simulink model "SpeedgoatCANOpen2Buses100us"  (R2018b)
settings: Solver=FixedStepDiscrete  StartTime=0.0  StopTime=inf  FixedStep=0.0001  RelTol=1e-3  EnableMultiTasking=on
libraries: slrtlib x6, speedgoatlib_IO691 x5, simulink x3, dspstat3 x2, cstblocks x1
(part 2 of 2)

== system SpeedgoatCANOpen2Buses100us/Speedgoat_TPDOs/CAN Bus Communication/CANOpen Slave Protocol Stack - CAN Bus #2 (B) ==
  C Caller : CCaller  FunctionName=CANOpenSlave_ProcessStack_APT  PortSpecificationStruct="%)30     .    ( D   8    (     @         %    \"     8    !     0         %  0 \"0    $    V    07)G3F%M90  4&]R=$YA;64 4V-O<&4     26YD97@     5'EP90      4VEZ90         .    ,     8    (    !          %    \"     $    $     0         0  0 <GA)1 X    P    !@    @    $          4    (     0    0    !         !  ! !R>$E$#@   #@    &    \"     0         !0    @    !    !0    $         $     4   !);G ...(+2763 chars)"
  CAN RX Wrapper : Subsystem
  CAN TX Wrapper : Subsystem
  wires:
  CAN RX Wrapper/3(DATA) -> C Caller/3
  C Caller/3 -> CAN TX Wrapper/3(DATA)
  CAN RX Wrapper/2(DLC) -> C Caller/2
  C Caller/1 -> CAN TX Wrapper/1(ID)
  CAN RX Wrapper/1(ID) -> C Caller/1
  C Caller/2 -> CAN TX Wrapper/2(DLC), CAN TX Wrapper/Enable

== system SpeedgoatCANOpen2Buses100us/Trike Application Layer/System_Control/BrakeControl ==
  Brake control [%] : Inport
  Amp2mAmp : Gain  Gain=1000
  Data Type Conversion : DataTypeConversion  OutDataTypeStr=uint16
  Gain1 : Gain  Gain=12.7
  Gain2 : Gain  Gain=-1
  Gain3 : Gain  Gain=0.00015625
  Saturation : Saturate  UpperLimit=0  LowerLimit=-1
  Saturation1 : Saturate  UpperLimit=10000  LowerLimit=3600
  Sum : Sum  Inputs=|+-
  offset : Constant  Value=3600
  Br CurrentRef [mA] : Outport
  wires:
  Saturation/1 -> Gain1/1
  Gain1/1 -> Amp2mAmp/1
  Brake control [%]/1 -> Data Type Conversion/1
  Gain2/1 -> Saturation/1
  Amp2mAmp/1 -> Br CurrentRef [mA]/1  "Br CurrentRef"
  Sum/1 -> Gain3/1
  offset/1 -> Sum/2
  Gain3/1 -> Gain2/1  "br_percent"
  Data Type Conversion/1 -> Saturation1/1
  Saturation1/1 -> Sum/1

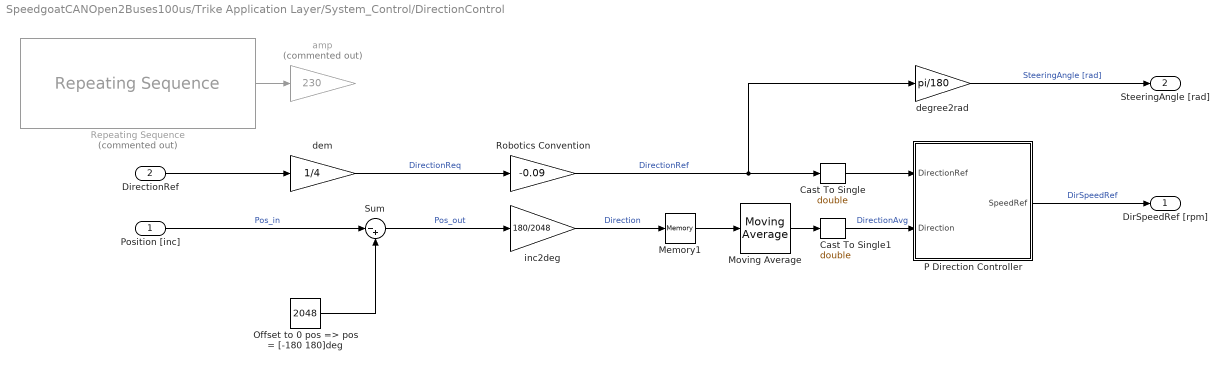
== system SpeedgoatCANOpen2Buses100us/Trike Application Layer/System_Control/DirectionControl ==
  Position [inc] : Inport
  DirectionRef : Inport  Port=2
  Cast To Single : DataTypeConversion  OutDataTypeStr=double
  Cast To Single1 : DataTypeConversion  OutDataTypeStr=double
  Memory1 : Memory  InheritSampleTime=on
  Moving Average : dspstat3/Moving Average  Method=Sliding window  ForgettingFactorPort=off  SpecifyWindowLength=on  WindowLength=1  ForgettingFactor=0.9  SimulateUsing=Code generation
  Offset to 0 pos => pos = [-180 180]deg : Constant  Value=2048
  P Direction Controller : MATLAB Function  TreatAsAtomicUnit=on  SystemSampleTime=5e-3
  Repeating Sequence : simulink/Sources/Repeating Sequence  Commented=on  rep_seq_t=[0 3 3.01 6 6.01 9 9.01 12]*5  rep_seq_y=[1 1 0 0 -1 -1 0 0]
  Robotics Convention : Gain  Gain=-0.09
  Sum : Sum  Inputs=|-+
  amp : Gain  Commented=on  Gain=230
  degree2rad : Gain  Gain=pi/180
  dem : Gain  Gain=1/4
  inc2deg : Gain  Gain=180/2048
  DirSpeedRef [rpm] : Outport
  SteeringAngle [rad] : Outport  Port=2
  wires:
  Memory1/1 -> Moving Average/1
  degree2rad/1 -> SteeringAngle [rad]/1  "SteeringAngle [rad]"
  inc2deg/1 -> Memory1/1  "Direction"
  DirectionRef/1 -> dem/1
  P Direction Controller/1(SpeedRef) -> DirSpeedRef [rpm]/1  "DirSpeedRef"
  Robotics Convention/1 -> Cast To Single/1, degree2rad/1  "DirectionRef"
  Cast To Single/1 -> P Direction Controller/1(DirectionRef)
  Cast To Single1/1 -> P Direction Controller/2(Direction)  "DirectionAvg"
  Position [inc]/1 -> Sum/1  "Pos_in"
  Sum/1 -> inc2deg/1  "Pos_out"
  Offset to 0 pos => pos = [-180 180]deg/1 -> Sum/2
  Moving Average/1 -> Cast To Single1/1
  Repeating Sequence/1 -> amp/1
  dem/1 -> Robotics Convention/1  "DirectionReq"

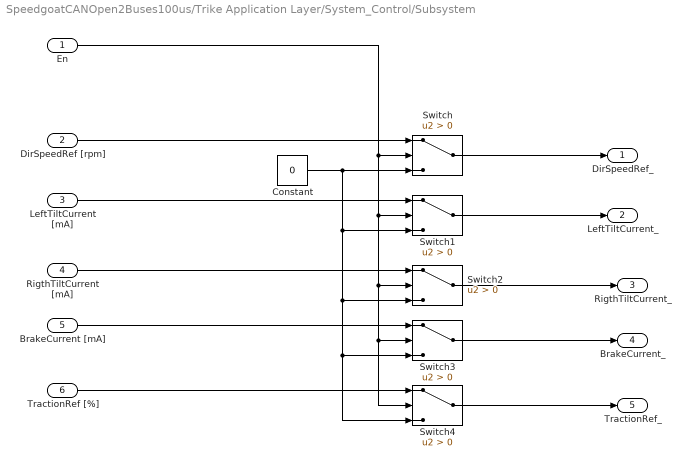
== system SpeedgoatCANOpen2Buses100us/Trike Application Layer/System_Control/Subsystem ==
  En : Inport
  DirSpeedRef [rpm] : Inport  Port=2
  LeftTiltCurrent [mA] : Inport  Port=3
  RigthTiltCurrent [mA] : Inport  Port=4
  BrakeCurrent [mA] : Inport  Port=5
  TractionRef [%] : Inport  Port=6
  Constant : Constant  Value=0
  Switch{,1..4} (5 alike) : Switch  Criteria=u2 > Threshold
  DirSpeedRef_ : Outport
  LeftTiltCurrent_ : Outport  Port=2
  RigthTiltCurrent_ : Outport  Port=3
  BrakeCurrent_ : Outport  Port=4
  TractionRef_ : Outport  Port=5
  wires:
  TractionRef [%]/1 -> Switch4/1
  Switch1/1 -> LeftTiltCurrent_/1
  Switch2/1 -> RigthTiltCurrent_/1
  En/1 -> Switch1/2, Switch2/2, Switch3/2, Switch4/2, Switch/2
  DirSpeedRef [rpm]/1 -> Switch/1
  LeftTiltCurrent [mA]/1 -> Switch1/1
  Constant/1 -> Switch3/3, Switch4/3, Switch2/3, Switch1/3, Switch/3
  Switch/1 -> DirSpeedRef_/1
  BrakeCurrent [mA]/1 -> Switch3/1
  Switch3/1 -> BrakeCurrent_/1
  Switch4/1 -> TractionRef_/1
  RigthTiltCurrent [mA]/1 -> Switch2/1

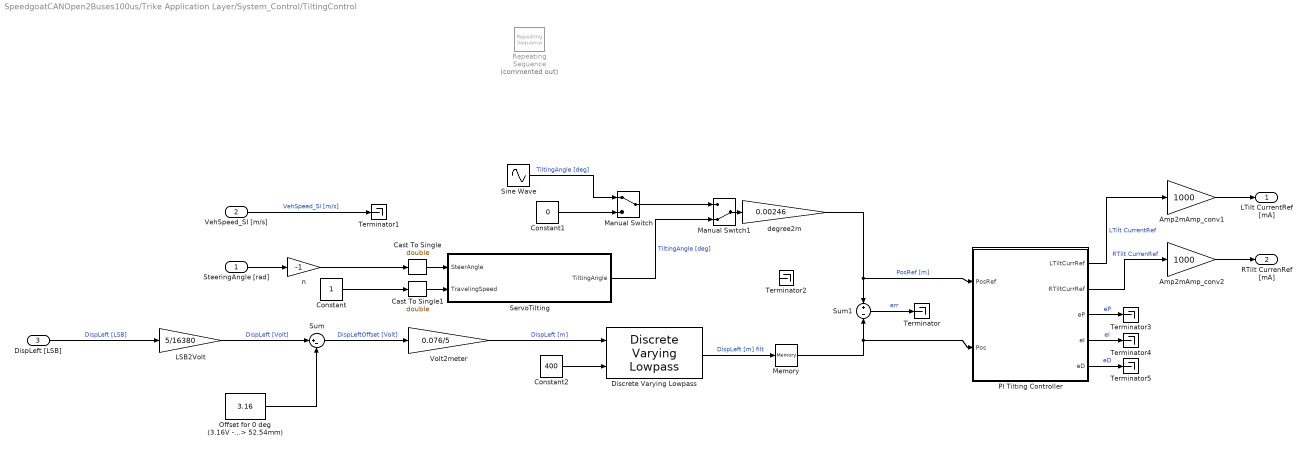
== system SpeedgoatCANOpen2Buses100us/Trike Application Layer/System_Control/TiltingControl ==
  SteeringAngle [rad] : Inport
  VehSpeed_SI [m/s] : Inport  Port=2
  DispLeft [LSB] : Inport  Port=3
  Amp2mAmp_conv1 : Gain  Gain=1000
  Amp2mAmp_conv2 : Gain  Gain=1000
  Cast To Single : DataTypeConversion  OutDataTypeStr=double
  Cast To Single1 : DataTypeConversion  OutDataTypeStr=double
  Constant : Constant
  Constant1 : Constant  Value=0
  Constant2 : Constant  Value=400
  Discrete Varying Lowpass : cstblocks/Linear Parameter Varying/Discrete Varying Lowpass  N=1  w0=0.5  Ts=0.0001
      settings: SourceProductName=Control System Toolbox  SourceProductBaseCode=CT
  LSB2Volt : Gain  Gain=5/16380
  Manual Switch : ManualSwitch
  Manual Switch1 : ManualSwitch  CurrentSetting=0
  Memory : Memory  InheritSampleTime=on
  "Offset for 0 deg (3.16V -> 52.54mm)" : Constant  Value=3.16
  PI Tilting Controller : MATLAB Function  TreatAsAtomicUnit=on  SystemSampleTime=5e-3
  Repeating Sequence : simulink/Sources/Repeating Sequence  Commented=on  rep_seq_t=[0 10 10.01 20 20.01 30 30.01 40] * 0.004  rep_seq_y=[1 1 -1 -1 1 1 -1 -1]
  ServoTilting : MATLAB Function  TreatAsAtomicUnit=on
      settings: MinAlgLoopOccurrences=on
  Sine Wave : Sin  Amplitude=2  Frequency=0.5  SampleTime=0
  Sum : Sum  Inputs=|+-
  Sum1 : Sum  Inputs=+-
  Terminator{,1..5} (6 alike) : Terminator
  Volt2meter : Gain  Gain=0.076/5
  degree2m : Gain  Gain=0.00246
  n : Gain  Gain=-1
  LTilt CurrentRef [mA] : Outport
  RTilt CurrenRef [mA] : Outport  Port=2
  wires:
  degree2m/1 -> Sum1/1, PI Tilting Controller/1(PosRef)  "PosRef [m]"
  Memory/1 -> PI Tilting Controller/2(Pos), Sum1/2
  Sine Wave/1 -> Manual Switch/1  "TiltingAngle [deg]"
  SteeringAngle [rad]/1 -> n/1
  Volt2meter/1 -> Discrete Varying Lowpass/1  "DispLeft [m]"
  PI Tilting Controller/2(RTiltCurrRef) -> Amp2mAmp_conv2/1  "RTilt CurrenRef"
  "Offset for 0 deg (3.16V -> 52.54mm)"/1 -> Sum/2
  PI Tilting Controller/1(LTiltCurrRef) -> Amp2mAmp_conv1/1  "LTilt CurrentRef"
  Constant/1 -> Cast To Single1/1
  Cast To Single/1 -> ServoTilting/1(SteerAngle)
  Cast To Single1/1 -> ServoTilting/2(TravelingSpeed)
  DispLeft [LSB]/1 -> LSB2Volt/1  "DispLeft [LSB]"
  Amp2mAmp_conv1/1 -> LTilt CurrentRef [mA]/1
  Amp2mAmp_conv2/1 -> RTilt CurrenRef [mA]/1
  Sum/1 -> Volt2meter/1  "DispLeftOffset [Volt]"
  Sum1/1 -> Terminator/1  "err"
  VehSpeed_SI [m/s]/1 -> Terminator1/1  "VehSpeed_SI [m/s]"
  Constant1/1 -> Manual Switch/2
  ServoTilting/1(TiltingAngle) -> Manual Switch1/2  "TiltingAngle [deg]"
  LSB2Volt/1 -> Sum/1  "DispLeft [Volt]"
  Discrete Varying Lowpass/1 -> Memory/1  "DispLeft [m] filt"
  Constant2/1 -> Discrete Varying Lowpass/2
  Manual Switch/1 -> Manual Switch1/1
  PI Tilting Controller/3(eP) -> Terminator3/1  "eP"
  PI Tilting Controller/4(eI) -> Terminator4/1  "eI"
  PI Tilting Controller/5(eD) -> Terminator5/1  "eD"
  Manual Switch1/1 -> degree2m/1
  n/1 -> Cast To Single/1

== system SpeedgoatCANOpen2Buses100us/Trike Application Layer/System_Control/TractionControl ==
  Traction Torque [%] : Inport
  SpeedRear_Fb : Inport  Port=2
  Abs : Abs
  Gain1 : Gain  Gain=1/10
  Gain2 : Gain  Gain=pi/30
  Terminator1 : Terminator
  WheelRadius : Gain  Gain=0.25
  m/s2Km/h : Gain  Gain=3.6
  VehSpeed_SI [m/s] : Outport
  TractionRef [%] : Outport  Port=2
  wires:
  Traction Torque [%]/1 -> Gain1/1
  Abs/1 -> TractionRef [%]/1  "TractionRef"
  WheelRadius/1 -> m/s2Km/h/1, VehSpeed_SI [m/s]/1  "VehSpeed_SI"
  SpeedRear_Fb/1 -> Gain2/1
  Gain2/1 -> WheelRadius/1  "SpeedRear_SI"
  m/s2Km/h/1 -> Terminator1/1  "VehSpeed_Km/h"
  Gain1/1 -> Abs/1

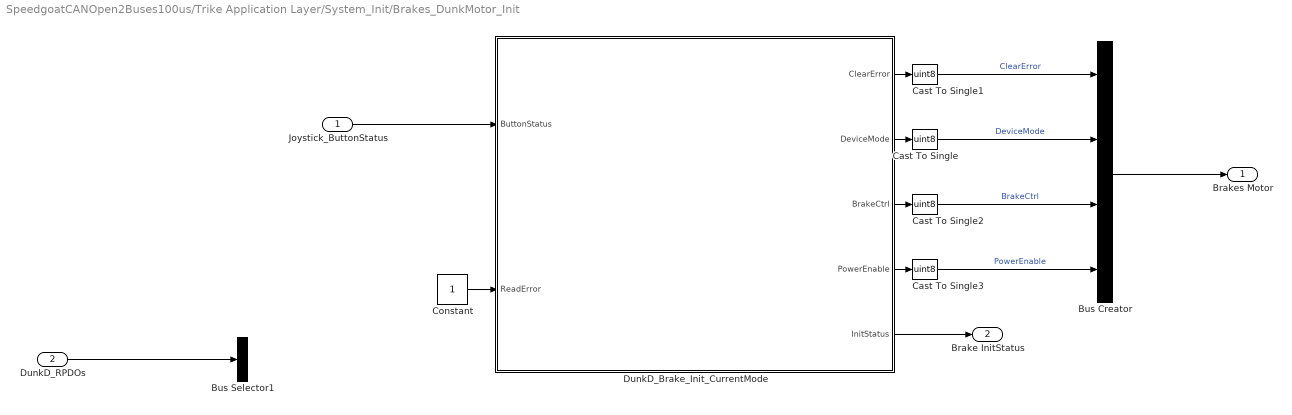
== system SpeedgoatCANOpen2Buses100us/Trike Application Layer/System_Init/Brakes_DunkMotor_Init ==
  Joystick_ButtonStatus : Inport
  DunkD_RPDOs : Inport  Port=2  OutDataTypeStr=Bus: Dunk_RPDOs
  Bus Creator : BusCreator  Inputs=4  OutDataTypeStr=Bus: Dunk_Init_TPDOs
  Bus Selector1 : BusSelector  OutputSignals=DunkD_ActualVelocity
  Cast To Single{,1..3} (4 alike) : DataTypeConversion  OutDataTypeStr=uint8
  Constant : Constant  OutDataTypeStr=single
  DunkD_Brake_Init_CurrentMode : Stateflow chart  TreatAsAtomicUnit=on
  Brakes Motor : Outport  OutDataTypeStr=Bus: Dunk_Init_TPDOs
  Brake InitStatus : Outport  Port=2
  wires:
  DunkD_RPDOs/1 -> Bus Selector1/1
  Bus Creator/1 -> Brakes Motor/1
  Cast To Single1/1 -> Bus Creator/1  "ClearError"
  Cast To Single/1 -> Bus Creator/2  "DeviceMode"
  Cast To Single2/1 -> Bus Creator/3  "BrakeCtrl"
  Cast To Single3/1 -> Bus Creator/4  "PowerEnable"
  DunkD_Brake_Init_CurrentMode/5(InitStatus) -> Brake InitStatus/1
  DunkD_Brake_Init_CurrentMode/1(ClearError) -> Cast To Single1/1
  Joystick_ButtonStatus/1 -> DunkD_Brake_Init_CurrentMode/1(ButtonStatus)
  DunkD_Brake_Init_CurrentMode/2(DeviceMode) -> Cast To Single/1
  DunkD_Brake_Init_CurrentMode/3(BrakeCtrl) -> Cast To Single2/1
  DunkD_Brake_Init_CurrentMode/4(PowerEnable) -> Cast To Single3/1
  Constant/1 -> DunkD_Brake_Init_CurrentMode/2(ReadError)

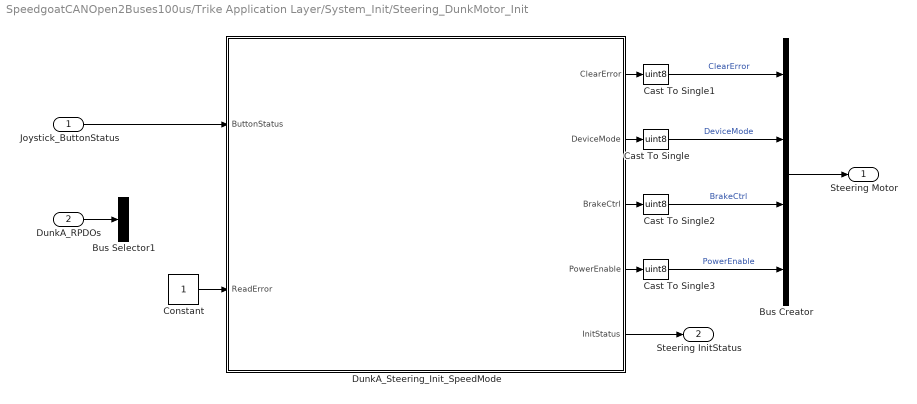
== system SpeedgoatCANOpen2Buses100us/Trike Application Layer/System_Init/Steering_DunkMotor_Init ==
  Joystick_ButtonStatus : Inport
  DunkA_RPDOs : Inport  Port=2  OutDataTypeStr=Bus: Dunk_RPDOs
  Bus Creator : BusCreator  Inputs=4  OutDataTypeStr=Bus: Dunk_Init_TPDOs
  Bus Selector1 : BusSelector  OutputSignals=DunkA_ActualVelocity
  Cast To Single{,1..3} (4 alike) : DataTypeConversion  OutDataTypeStr=uint8
  Constant : Constant  OutDataTypeStr=single
  DunkA_Steering_Init_SpeedMode : Stateflow chart  TreatAsAtomicUnit=on
  Steering Motor : Outport  OutDataTypeStr=Bus: Dunk_Init_TPDOs
  Steering InitStatus : Outport  Port=2
  wires:
  Bus Creator/1 -> Steering Motor/1
  DunkA_RPDOs/1 -> Bus Selector1/1
  DunkA_Steering_Init_SpeedMode/1(ClearError) -> Cast To Single1/1
  DunkA_Steering_Init_SpeedMode/2(DeviceMode) -> Cast To Single/1
  DunkA_Steering_Init_SpeedMode/3(BrakeCtrl) -> Cast To Single2/1
  DunkA_Steering_Init_SpeedMode/4(PowerEnable) -> Cast To Single3/1
  Joystick_ButtonStatus/1 -> DunkA_Steering_Init_SpeedMode/1(ButtonStatus)
  Constant/1 -> DunkA_Steering_Init_SpeedMode/2(ReadError)
  Cast To Single1/1 -> Bus Creator/1  "ClearError"
  Cast To Single/1 -> Bus Creator/2  "DeviceMode"
  Cast To Single2/1 -> Bus Creator/3  "BrakeCtrl"
  Cast To Single3/1 -> Bus Creator/4  "PowerEnable"
  DunkA_Steering_Init_SpeedMode/5(InitStatus) -> Steering InitStatus/1

== system SpeedgoatCANOpen2Buses100us/Trike Application Layer/System_Init/Subsystem ==
  Steering InitStatus : Inport
  TiltLeft InitStatus : Inport  Port=2
  TiltRight InitStatus : Inport  Port=3
  Brake InitStatus : Inport  Port=4
  MiniMaster_Enable : Inport  Port=5
  Compare To Constant : simulink/Logic and Bit Operations/Compare To Constant  relop===  const=5  OutDataTypeStr=boolean
  Sum : Sum  Inputs=+++++
  EnableControl : Outport
  wires:
  Sum/1 -> Compare To Constant/1
  Brake InitStatus/1 -> Sum/4  "Brake_InitStatus"
  Steering InitStatus/1 -> Sum/1  "Steering_InitStatus"
  TiltRight InitStatus/1 -> Sum/3  "TiltRight_InitStatus"
  TiltLeft InitStatus/1 -> Sum/2  "TiltLeft_InitStatus"
  MiniMaster_Enable/1 -> Sum/5  "MiniMaster_Enable"
  Compare To Constant/1 -> EnableControl/1  "EnableControl"

== system SpeedgoatCANOpen2Buses100us/Trike Application Layer/System_Init/TiltingLeft_DunkMotor_Init ==
  Joystick_ButtonStatus : Inport
  DunkB_RPDOs : Inport  Port=2  OutDataTypeStr=Bus: Dunk_RPDOs
  Bus Creator : BusCreator  Inputs=4  OutDataTypeStr=Bus: Dunk_Init_TPDOs
  Bus Selector1 : BusSelector  OutputSignals=DunkB_ActualVelocity
  Cast To Single{,1..3} (4 alike) : DataTypeConversion  OutDataTypeStr=uint8
  Constant : Constant  OutDataTypeStr=single
  DunkB_TiltLeft_Init_CurrentMode : Stateflow chart  TreatAsAtomicUnit=on
  TiltLeft Motor : Outport  OutDataTypeStr=Bus: Dunk_Init_TPDOs
  TiltLeft InitStatus : Outport  Port=2
  wires:
  DunkB_RPDOs/1 -> Bus Selector1/1
  Bus Creator/1 -> TiltLeft Motor/1
  DunkB_TiltLeft_Init_CurrentMode/5(InitStatus) -> TiltLeft InitStatus/1
  Cast To Single/1 -> Bus Creator/2  "DeviceMode"
  Constant/1 -> DunkB_TiltLeft_Init_CurrentMode/2(ReadError)
  Cast To Single2/1 -> Bus Creator/3  "BrakeCtrl"
  DunkB_TiltLeft_Init_CurrentMode/4(PowerEnable) -> Cast To Single3/1
  DunkB_TiltLeft_Init_CurrentMode/3(BrakeCtrl) -> Cast To Single2/1
  Cast To Single3/1 -> Bus Creator/4  "PowerEnable"
  DunkB_TiltLeft_Init_CurrentMode/2(DeviceMode) -> Cast To Single/1
  Cast To Single1/1 -> Bus Creator/1  "ClearError"
  DunkB_TiltLeft_Init_CurrentMode/1(ClearError) -> Cast To Single1/1
  Joystick_ButtonStatus/1 -> DunkB_TiltLeft_Init_CurrentMode/1(ButtonStatus)

== system SpeedgoatCANOpen2Buses100us/Trike Application Layer/System_Init/TiltingRight_DunkMotor_Init ==
  Joystick_ButtonStatus : Inport
  DunkC_RPDOs : Inport  Port=2  OutDataTypeStr=Bus: Dunk_RPDOs
  Bus Creator : BusCreator  Inputs=4  OutDataTypeStr=Bus: Dunk_Init_TPDOs
  Bus Selector1 : BusSelector  OutputSignals=DunkC_ActualVelocity
  Cast To Single{,1..3} (4 alike) : DataTypeConversion  OutDataTypeStr=uint8
  Constant : Constant  OutDataTypeStr=single
  DunkC_TiltRight_Init_CurrentMode : Stateflow chart  TreatAsAtomicUnit=on
  TiltRight Motor : Outport  OutDataTypeStr=Bus: Dunk_Init_TPDOs
  TiltRight InitStatus : Outport  Port=2
  wires:
  Bus Creator/1 -> TiltRight Motor/1
  DunkC_RPDOs/1 -> Bus Selector1/1
  Cast To Single1/1 -> Bus Creator/1  "ClearError"
  Cast To Single/1 -> Bus Creator/2  "DeviceMode"
  Cast To Single2/1 -> Bus Creator/3  "BrakeCtrl"
  Cast To Single3/1 -> Bus Creator/4  "PowerEnable"
  DunkC_TiltRight_Init_CurrentMode/5(InitStatus) -> TiltRight InitStatus/1
  DunkC_TiltRight_Init_CurrentMode/1(ClearError) -> Cast To Single1/1
  Joystick_ButtonStatus/1 -> DunkC_TiltRight_Init_CurrentMode/1(ButtonStatus)
  DunkC_TiltRight_Init_CurrentMode/2(DeviceMode) -> Cast To Single/1
  DunkC_TiltRight_Init_CurrentMode/3(BrakeCtrl) -> Cast To Single2/1
  DunkC_TiltRight_Init_CurrentMode/4(PowerEnable) -> Cast To Single3/1
  Constant/1 -> DunkC_TiltRight_Init_CurrentMode/2(ReadError)

== system SpeedgoatCANOpen2Buses100us/Speedgoat_TPDOs/CAN Bus Communication/CANOpen Slave Protocol Stack - CAN Bus #1 (A)/CAN RX Wrapper ==
  CAN Read : speedgoatlib_IO691/CAN Read  id=1  ts=Ts  channel=1  messageType=RAW  canType=CAN (HS)  initValues=[691 1 0.0001 0 2 1]
      settings: SourceProductName=Simulink Real-Time: Speedgoat Library
  Constant : Constant  Commented=on  Value=0  OutDataTypeStr=Inherit: Inherit via back propagation
  Switch : Switch  Criteria=u2 > Threshold
  Terminator : Terminator
  Terminator1 : Terminator
  ID : Outport
  DLC : Outport  Port=2
  DATA : Outport  Port=3
  wires:
  CAN Read/4 -> Switch/3
  CAN Read/5 -> Terminator1/1
  Switch/1 -> DLC/1
  CAN Read/2 -> ID/1
  CAN Read/3 -> Switch/2
  CAN Read/6 -> DATA/1
  Constant/1 -> Switch/1
  CAN Read/1 -> Terminator/1

== system SpeedgoatCANOpen2Buses100us/Speedgoat_TPDOs/CAN Bus Communication/CANOpen Slave Protocol Stack - CAN Bus #1 (A)/CAN TX Wrapper ==
  ID : Inport
  DLC : Inport  Port=2
  DATA : Inport  Port=3
  Enable : EnablePort
  CAN Write : speedgoatlib_IO691/CAN Write  id=1  ts=Ts  channel=1  messageType=RAW  enableStatusPort=off  canType=CAN (HS)  initValues=[691 1 0.0001 0 2 1 0]
      settings: SourceProductName=Simulink Real-Time: Speedgoat Library
  Constant : Constant  Value=0  OutDataTypeStr=Inherit: Inherit via back propagation
  wires:
  ID/1 -> CAN Write/1
  DATA/1 -> CAN Write/4
  DLC/1 -> CAN Write/3
  Constant/1 -> CAN Write/2

== system SpeedgoatCANOpen2Buses100us/Speedgoat_TPDOs/CAN Bus Communication/CANOpen Slave Protocol Stack - CAN Bus #2 (B)/CAN RX Wrapper ==
  CAN Read : speedgoatlib_IO691/CAN Read  id=1  ts=Ts  channel=2  messageType=RAW  canType=CAN (HS)  initValues=[691 1 0.0001 1 2 1]
      settings: SourceProductName=Simulink Real-Time: Speedgoat Library
  Constant : Constant  Commented=on  Value=0  OutDataTypeStr=Inherit: Inherit via back propagation
  Switch : Switch  Criteria=u2 > Threshold
  Terminator : Terminator
  Terminator1 : Terminator
  ID : Outport
  DLC : Outport  Port=2
  DATA : Outport  Port=3
  wires:
  CAN Read/1 -> Terminator/1
  Constant/1 -> Switch/1
  CAN Read/6 -> DATA/1
  CAN Read/3 -> Switch/2
  CAN Read/2 -> ID/1
  Switch/1 -> DLC/1
  CAN Read/5 -> Terminator1/1
  CAN Read/4 -> Switch/3

== system SpeedgoatCANOpen2Buses100us/Speedgoat_TPDOs/CAN Bus Communication/CANOpen Slave Protocol Stack - CAN Bus #2 (B)/CAN TX Wrapper ==
  ID : Inport
  DLC : Inport  Port=2
  DATA : Inport  Port=3
  Enable : EnablePort
  CAN Write : speedgoatlib_IO691/CAN Write  id=1  ts=Ts  channel=2  messageType=RAW  enableStatusPort=off  canType=CAN (HS)  initValues=[691 1 0.0001 1 2 1 0]
      settings: SourceProductName=Simulink Real-Time: Speedgoat Library
  Constant : Constant  Value=0  OutDataTypeStr=Inherit: Inherit via back propagation
  wires:
  Constant/1 -> CAN Write/2
  DLC/1 -> CAN Write/3
  DATA/1 -> CAN Write/4
  ID/1 -> CAN Write/1

== stateflow chart SpeedgoatCANOpen2Buses100us/Trike Application Layer/System_Init/TiltingLeft_DunkMotor_Init/DunkB_TiltLeft_Init_CurrentMode ==
  state Init
    entry:
    ClearError       = 0;
    DeviceMode   = 0;
    BrakeCtrl        = 0;
    PowerEnable = 0;
    aux                 = 0;
    InitStatus        = 0;
  state Clear_Error
    du:
    ClearError = 1;
    aux=aux+1;
    InitStatus = 0;
  state Wait
    en:
    BrakeCtrl = 2;
    aux = 0;
    InitStatus = 0;
  state SetCurrentMode
    du:
    DeviceMode  = 2;
    PowerEnable = 1;
    InitStatus       = 1;
  (default) -> Init
  Init -> Clear_Error : [ButtonStatus == 1 || ReadError ~= 1]
  Wait -> Init [order 3] : [ReadError ~= 1]
  SetCurrentMode -> Init : [ReadError ~= 1]
  Clear_Error -> Wait : [aux>2000]
  Wait -> Wait [order 1] : [ButtonStatus==0 && ReadError == 1]
  Wait -> SetCurrentMode [order 2] : [ButtonStatus==2 && ReadError == 1]
  data: ButtonStatus input single; ClearError output single; DeviceMode output single; BrakeCtrl output single; ReadError input single; aux2 local single; aux local single; PowerEnable output single; InitStatus output single

== stateflow chart SpeedgoatCANOpen2Buses100us/Trike Application Layer/System_Init/TiltingRight_DunkMotor_Init/DunkC_TiltRight_Init_CurrentMode ==
  state Init
    entry:
    ClearError       = 0;
    DeviceMode   = 0;
    BrakeCtrl        = 0;
    PowerEnable = 0;
    aux                 = 0;
    InitStatus        = 0;
  state Clear_Error
    du:
    ClearError = 1;
    aux=aux+1;
    InitStatus = 0;
  state Wait
    en:
    BrakeCtrl = 2;
    aux = 0;
    InitStatus = 0;
  state SetCurrentMode
    du:
    DeviceMode  = 2;
    PowerEnable = 1;
    InitStatus       = 1;
  (default) -> Init
  Init -> Clear_Error : [ButtonStatus == 1 || ReadError ~= 1]
  Wait -> Init [order 3] : [ReadError ~= 1]
  SetCurrentMode -> Init : [ReadError ~= 1]
  Clear_Error -> Wait : [aux>2000]
  Wait -> Wait [order 1] : [ButtonStatus==0 && ReadError == 1]
  Wait -> SetCurrentMode [order 2] : [ButtonStatus==2 && ReadError == 1]
  data: ButtonStatus input single; ClearError output single; DeviceMode output single; BrakeCtrl output single; ReadError input single; aux2 local single; aux local single; PowerEnable output single; InitStatus output single

== stateflow chart SpeedgoatCANOpen2Buses100us/Trike Application Layer/System_Init/Brakes_DunkMotor_Init/DunkD_Brake_Init_CurrentMode ==
  state Init
    entry:
    ClearError       = 0;
    DeviceMode   = 0;
    BrakeCtrl        = 0;
    PowerEnable = 0;
    aux                 = 0;
    InitStatus        = 0;
  state Clear_Error
    du:
    ClearError = 1;
    aux=aux+1;
    InitStatus = 0;
  state Wait
    en:
    BrakeCtrl = 2;
    aux = 0;
    InitStatus = 0;
  state SetCurrentMode
    du:
    DeviceMode  = 2;
    PowerEnable = 1;
    InitStatus       = 1;
  (default) -> Init
  Init -> Clear_Error : [ButtonStatus == 1 || ReadError ~= 1]
  Wait -> Init [order 3] : [ReadError ~= 1]
  SetCurrentMode -> Init : [ReadError ~= 1]
  Clear_Error -> Wait : [aux>2000]
  Wait -> Wait [order 1] : [ButtonStatus==0 && ReadError == 1]
  Wait -> SetCurrentMode [order 2] : [ButtonStatus==2 && ReadError == 1]
  data: ButtonStatus input single; ClearError output single; DeviceMode output single; BrakeCtrl output single; ReadError input single; aux2 local single; aux local single; PowerEnable output single; InitStatus output single

== stateflow chart SpeedgoatCANOpen2Buses100us/Trike Application Layer/System_Init/EnableCtrl ==
  state Init
    du:
    Enable    =  0;
  state Enable_Control
    du:
    Enable    =  1;
  (default) -> Init
  Init -> Enable_Control : [ButtonStatus == 6 ]
  Enable_Control -> Init : [ButtonStatus == 7 ]
  data: ButtonStatus input single; Enable output single

== matlab function SpeedgoatCANOpen2Buses100us/Trike Application Layer/System_Control/DirectionControl/P Direction Controller ==
  data: DirectionRef input; SpeedRef output; Direction input
function SpeedRef  = fcn(DirectionRef,Direction)


if (DirectionRef>90)
    DirectionRef=90;
end
if (DirectionRef<-90)
    DirectionRef=-90;
end
err = DirectionRef - Direction;

Kp = 70;

SpeedRef = Kp * err;  


end

== matlab function SpeedgoatCANOpen2Buses100us/Trike Application Layer/System_Control/TiltingControl/PI Tilting Controller ==
  data: PosRef input; LTiltCurrRef output; Pos input; RTiltCurrRef output; eP output; eI output; eD output
function [LTiltCurrRef, RTiltCurrRef,eP,eI,eD] = fcn(PosRef,Pos)
persistent uk1 ek1 ek2
if (isempty(uk1))
    uk1 = 0;
    ek1 = 0;
    ek2 = 0;
end

% +/- 0.076 m
pos_lim = 0.02;
imax = 5;

Kp = 1000;
Ki = 1;
Kd = 800;

if (PosRef > pos_lim)
    PosRef = pos_lim;
end
if (PosRef <- pos_lim)
   PosRef = -pos_lim;
end

e = PosRef - Pos;


Du = Ki * e + Kp * (e - ek1) + Kd * (e - 2*ek1 + ek2);

eP = Kp*(e - ek1) ;
eI =  Ki*e ;
eD = Kd*(e - 2*ek1 + ek2);


u = uk1 + Du;

if (u >imax)
    u = imax;
end
if (u<-imax)
    u=-imax;
end

LTiltCurrRef =  u;
RTiltCurrRef =  -u;
uk1 = u;
ek1 = e;
ek2 = ek1;

== matlab function SpeedgoatCANOpen2Buses100us/Trike Application Layer/System_Control/TiltingControl/ServoTilting ==
  data: SteerAngle input; TravelingSpeed input; TiltingAngle output
function TiltingAngle  = CalcTiltAngle(SteerAngle,TravelingSpeed)
%SteerAngle [rad]
%TravelingSpeed [m/s]
L = 1.025;
g = 9.81;
TiltingAngle = atan(TravelingSpeed^2/(L*g)*sin(SteerAngle));
TiltingAngle = TiltingAngle *180/pi;
% TiltingAngle [deg]

== stateflow chart SpeedgoatCANOpen2Buses100us/Trike Application Layer/System_Init/Steering_DunkMotor_Init/DunkA_Steering_Init_SpeedMode ==
  state Init
    entry:
    ClearError       = 0;
    DeviceMode   = 0;
    BrakeCtrl        = 0;
    PowerEnable = 0;
    aux                 = 0;
    InitStatus        = 0;
  state Clear_Error
    du:
    ClearError = 1;
    aux=aux+1;
    InitStatus = 0;
  state Wait
    en:
    BrakeCtrl = 2;
    aux = 0;
    InitStatus = 0;
  state SetCurrentMode
    du:
    DeviceMode  = 3; % SpeedMode
    PowerEnable = 1;
    InitStatus       = 1;
  (default) -> Init
  Init -> Clear_Error : [ButtonStatus == 1 || ReadError ~= 1]
  Wait -> Init [order 3] : [ReadError ~= 1]
  SetCurrentMode -> Init : [ReadError ~= 1]
  Clear_Error -> Wait : [aux>2000]
  Wait -> Wait [order 1] : [ButtonStatus==0 && ReadError == 1]
  Wait -> SetCurrentMode [order 2] : [ButtonStatus==2 && ReadError == 1]
  data: ButtonStatus input single; ClearError output single; DeviceMode output single; BrakeCtrl output single; ReadError input single; aux2 local single; aux local single; PowerEnable output single; InitStatus output single

== matlab function SpeedgoatCANOpen2Buses100us/Trike Application Layer/System_Init/MATLAB Function ==
  data: ButtonStatus input; button output
function button = JoystickButtonStatus(ButtonStatus)
aux = 0;
switch (ButtonStatus)
    case 1
        aux = 1;
    case 2
        aux = 2;
    case 4
        aux = 3;
    case 8
        aux = 4;
    case 16
        aux = 5;
    case 32
        aux = 6; 
    case 64
        aux = 7;
    case 128 
        aux = 8;
    otherwise
        aux = 0;
end
button =aux;

== matlab function SpeedgoatCANOpen2Buses100us/Trike Application Layer/Subsystem1/HeartBeatgenerator ==
  data: HB output
function HB = HBGenerator
persistent tact Heartbeat
if (isempty(Heartbeat))
    Heartbeat = 0;
    tact = 0;
end
tact=tact+1;
if (tact>10)
    tact=0;
    Heartbeat=Heartbeat+1;
    if (Heartbeat>127)
        Heartbeat = 0;    
    end
end
HB = Heartbeat;

== matlab function SpeedgoatCANOpen2Buses100us/Trike Application Layer/System_Init/MATLAB Function1 ==
  data: ButtonStatus input; Byte0 output; LongCmd input
function Byte0 = TractionCtrl(ButtonStatus, LongCmd)
Direction =0;
if (ButtonStatus==8)
    if(LongCmd>0)
        Direction = 4;
    elseif (LongCmd<0)
        Direction = 8;
    end
 end
Byte0 =160+Direction;
